simulink model "mBraccioHWblocks"  (R2021a)
settings: Solver=FixedStepAuto  StartTime=0.0  StopTime=inf  RelTol=1e-3  EnableMultiTasking=on
undefined symbols (not defined in the file): adHome5rad, adHome6deg, adHome6rad, adJointRanges, adLinkLenghts
libraries: arduinolib x17, aerolibconvert2 x3
settings Model: SILPILModeSetting=veronly  ExtModeTrigDuration=2  Creator=angelo  LastModifiedBy=angelo
settings OptimizationCC: EnhancedBackFolding=on  PassReuseOutputArgsAs=Individual arguments  ZeroExternalMemoryAtStartup=off  ZeroInternalMemoryAtStartup=off  MaxStackSize=64  OptimizeBlockOrder=speed  DifferentSizesBufferReuse=on  OptimizationCustomize=off  EfficientTunableParamExpr=on
settings DebuggingCC: ParameterTunabilityLossMsg=error
settings HardwareCC: ProdBitPerInt=16  ProdBitPerPointer=16  ProdBitPerSizeT=16  ProdBitPerPtrDiffT=16  ProdLargestAtomicFloat=None  ProdWordSize=8  ProdHWDeviceType=Atmel->AVR
settings SFSimCC: MATLABDynamicMemAlloc=off
settings RTWCC: SystemTargetFile=ert.tlc  HardwareBoard=Arduino Mega 2560  TemplateMakefile=ert_default_tmf  Toolchain=Arduino AVR  BuildConfiguration=Faster Runs
settings CodeAppCC: ForceParamTrailComments=on  IgnoreCustomStorageClasses=off  OperatorAnnotations=on  SimulinkDataObjDesc=on  SFDataObjDesc=on  InsertBlockDesc=on
settings ERTTargetCC: SupportContinuousTime=on  SupportVariableSizeSignals=on  ExtModeStaticAllocSize=2048

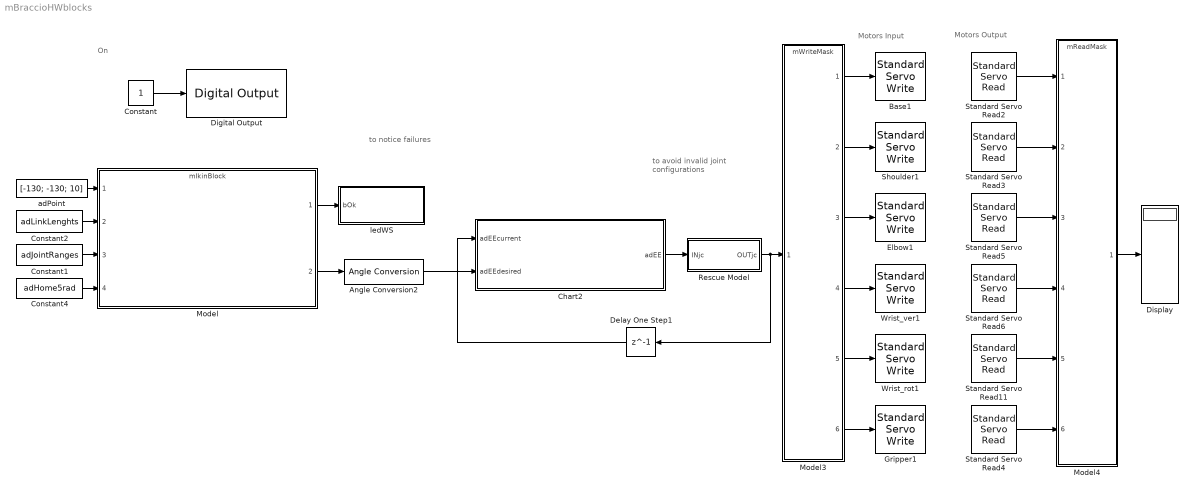
== system mBraccioHWblocks ==
  note: to avoid invalid joint configurations
  note: to notice failures
  note: Motors Output
  note: Motors Input
  note: On
  Angle Conversion2 : aerolibconvert2/Angle Conversion  IU=rad  OU=deg
  Base1 : arduinolib/Standard Servo Write  pinNumber=11  ServoIndex=0  blockPlatform=ARDUINO
  Chart2 : Stateflow chart  TreatAsAtomicUnit=on  SystemSampleTime=0.02
  Constant : Constant
  Constant1 : Constant  Value=adJointRanges
  Constant2 : Constant  Value=adLinkLenghts
  Constant4 : Constant  Value=adHome5rad
  Delay One Step1 : Delay  DelayLength=1  InitialCondition=adHome6deg
  Digital Output : arduinolib/Digital Output  pinNumber=12  Direction=output  blockPlatform=arduino
  Display : Display
  Elbow1 : arduinolib/Standard Servo Write  pinNumber=9  ServoIndex=1  blockPlatform=ARDUINO
  Gripper1 : arduinolib/Standard Servo Write  pinNumber=3  ServoIndex=2  blockPlatform=ARDUINO
  Model : ModelReference  ModelNameDialog=mIkinBlock.slx  SimulationMode=Normal  ModelReferenceVersion=1.87
  Model3 : ModelReference  ModelNameDialog=mWriteMask.slx  SimulationMode=Normal  ModelReferenceVersion=1.6
  Model4 : ModelReference  ModelNameDialog=mReadMask.slx  SimulationMode=Normal  ModelReferenceVersion=1.7
  Rescue Model : Subsystem
  Shoulder1 : arduinolib/Standard Servo Write  pinNumber=10  ServoIndex=3  blockPlatform=ARDUINO
  Standard Servo Read11 : arduinolib/Standard Servo Read  pinNumber=5  SampleTime=0.02  ServoIndex=4  blockPlatform=ARDUINO
      settings: SourceProductBaseCode=ARDUINO
  Standard Servo Read2 : arduinolib/Standard Servo Read  pinNumber=11  SampleTime=0.02  ServoIndex=0  blockPlatform=ARDUINO
      settings: SourceProductBaseCode=ARDUINO
  Standard Servo Read3 : arduinolib/Standard Servo Read  pinNumber=10  SampleTime=0.02  ServoIndex=3  blockPlatform=ARDUINO
      settings: SourceProductBaseCode=ARDUINO
  Standard Servo Read4 : arduinolib/Standard Servo Read  pinNumber=3  SampleTime=0.02  ServoIndex=2  blockPlatform=ARDUINO
      settings: SourceProductBaseCode=ARDUINO
  Standard Servo Read5 : arduinolib/Standard Servo Read  pinNumber=9  SampleTime=0.02  ServoIndex=1  blockPlatform=ARDUINO
      settings: SourceProductBaseCode=ARDUINO
  Standard Servo Read6 : arduinolib/Standard Servo Read  pinNumber=6  SampleTime=0.02  ServoIndex=5  blockPlatform=ARDUINO
      settings: SourceProductBaseCode=ARDUINO
  Wrist_rot1 : arduinolib/Standard Servo Write  pinNumber=5  ServoIndex=4  blockPlatform=ARDUINO
  Wrist_ver1 : arduinolib/Standard Servo Write  pinNumber=6  ServoIndex=5  blockPlatform=ARDUINO
  adPoint : Constant  Value=[-130; -130; 10]
  ledWS : Subsystem  TreatAsAtomicUnit=on
  wires:
  Rescue Model/1(OUTjc) -> Delay One Step1/1, Model3/1
  Model3/5 -> Wrist_rot1/1
  Constant1/1 -> Model/3
  Constant2/1 -> Model/2
  Model3/6 -> Gripper1/1
  Model/2 -> Angle Conversion2/1
  Standard Servo Read5/1 -> Model4/3
  Model/1 -> ledWS/1(bOk)
  Model3/3 -> Elbow1/1
  Standard Servo Read11/1 -> Model4/5
  Standard Servo Read6/1 -> Model4/4
  Angle Conversion2/1 -> Chart2/2(adEEdesired)
  Standard Servo Read3/1 -> Model4/2
  Model3/4 -> Wrist_ver1/1
  Standard Servo Read4/1 -> Model4/6
  Constant4/1 -> Model/4
  Delay One Step1/1 -> Chart2/1(adEEcurrent)
  Chart2/1(adEE) -> Rescue Model/1(INjc)
  Model3/1 -> Base1/1
  Standard Servo Read2/1 -> Model4/1
  Model3/2 -> Shoulder1/1
  Constant/1 -> Digital Output/1
  adPoint/1 -> Model/1
  Model4/1 -> Display/1

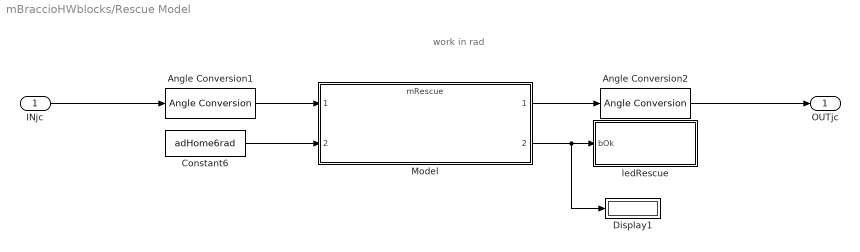
== system mBraccioHWblocks/Rescue Model ==
  note: work in rad
  INjc : Inport
  Angle Conversion1 : aerolibconvert2/Angle Conversion  IU=deg  OU=rad
  Angle Conversion2 : aerolibconvert2/Angle Conversion  IU=rad  OU=deg
  Constant6 : Constant  Value=adHome6rad
  Display1 : Display
  Model : ModelReference  ModelNameDialog=mRescue.slx  SimulationMode=Normal  ModelReferenceVersion=1.31
  ledRescue : Subsystem  TreatAsAtomicUnit=on
  OUTjc : Outport
  wires:
  Constant6/1 -> Model/2
  Angle Conversion1/1 -> Model/1
  INjc/1 -> Angle Conversion1/1
  Model/1 -> Angle Conversion2/1
  Angle Conversion2/1 -> OUTjc/1
  Model/2 -> Display1/1, ledRescue/1(bOk)

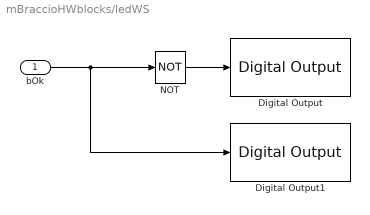
== system mBraccioHWblocks/ledWS ==
  bOk : Inport
  Digital Output : arduinolib/Digital Output  pinNumber=7  Direction=output  blockPlatform=arduino
  Digital Output1 : arduinolib/Digital Output  pinNumber=8  Direction=output  blockPlatform=arduino
  NOT : Logic  Operator=NOT  IconShape=distinctive  AllPortsSameDT=off  OutDataTypeStr=boolean
  wires:
  NOT/1 -> Digital Output/1
  bOk/1 -> Digital Output1/1, NOT/1

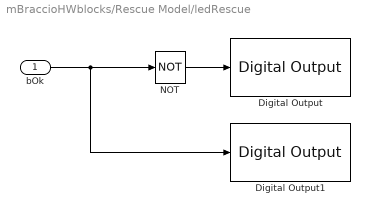
== system mBraccioHWblocks/Rescue Model/ledRescue ==
  bOk : Inport
  Digital Output : arduinolib/Digital Output  pinNumber=2  Direction=output  blockPlatform=arduino
  Digital Output1 : arduinolib/Digital Output  pinNumber=4  Direction=output  blockPlatform=arduino
  NOT : Logic  Operator=NOT  IconShape=distinctive  AllPortsSameDT=off  OutDataTypeStr=boolean
  wires:
  bOk/1 -> NOT/1, Digital Output1/1
  NOT/1 -> Digital Output/1

== stateflow chart mBraccioHWblocks/Chart2 ==
  settings: executeAtInitialization=1
  state First
    during:
    adEE = [
    nextStep(adEEcurrent(1), adEEdesired(1));
    nextStep(adEEcurrent(2), adEEdesired(2));
    nextStep(adEEcurrent(3), adEEdesired(3));
    nextStep(adEEcurrent(4), adEEdesired(4));
    nextStep(adEEcurrent(5), adEEdesired(5));
    nextStep(adEEcurrent(6), adEEdesired(6)) ];
  (default) -> First
  data: current function_input; desired function_input; v function_output; adEEcurrent input; adEE output; adEEdesired input
  function v = nextStep(current, desired):
    | function v = nextStep(current, desired)
    | if (current < desired)
    |     current = current + 1;
    | end
    | 
    | if (current > desired)
    |     current = current - 1;
    | end
    | 
    | v = current;
    | end
